simulink model "IMPLICIT_1ODE_EX6_sim"  (Simulink 8.0)
settings: Solver=ode45  StartTime=0.0  StopTime=130  RelTol=1e-3  AbsTol=1e-5
settings Model: Creator=David  LastModifiedBy=David
settings SolverCC: ZeroCrossControl=EnableAll

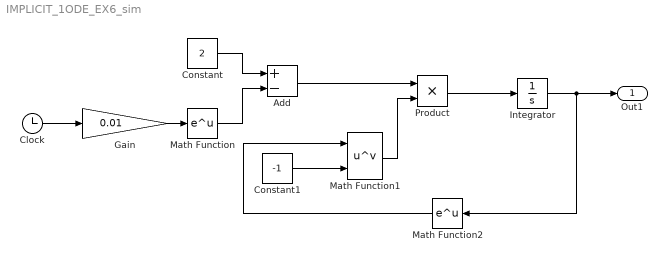
== system IMPLICIT_1ODE_EX6_sim ==
  Add : Sum  Inputs=+-
  Clock : Clock
  Constant : Constant  Value=2
  Constant1 : Constant  Value=-1
  Gain : Gain  Gain=0.01
  Integrator : Integrator  InitialCondition=2
  Math Function : Math  SaturateOnIntegerOverflow=on
  Math Function1 : Math  Operator=pow  SaturateOnIntegerOverflow=on
  Math Function2 : Math  SaturateOnIntegerOverflow=on
  Product : Product  RndMeth=Zero
  Out1 : Outport
  wires:
  Clock/1 -> Gain/1
  Gain/1 -> Math Function/1
  Constant/1 -> Add/1
  Math Function/1 -> Add/2
  Add/1 -> Product/1
  Product/1 -> Integrator/1
  Integrator/1 -> Out1/1, Math Function2/1
  Math Function1/1 -> Product/2
  Math Function2/1 -> Math Function1/1
  Constant1/1 -> Math Function1/2
